simulink model "testbench_stateflow_20b"  (R2020b)
settings: Solver=VariableStepAuto  StartTime=0.0  StopTime=10  FixedStep=0.01  RelTol=1e-3  EnableMultiTasking=on
libraries: simulink x5
settings Model: Creator=Schneider  LastModifiedBy=60251
settings DataIOCC: LimitDataPoints=on  ReturnWorkspaceOutputs=off
settings OptimizationCC: LifeSpan=inf
settings DebuggingCC: AllowSymbolicDim=off  SFUnexpectedBacktrackingDiag=warning  SFNoUnconditionalDefaultTransitionDiag=warning  SFExecutionAtInitializationDiag=none  ArithmeticOperatorsInVariantConditions=warning
settings ModelReferenceCC: PropagateSignalLabelsOutOfModel=off
settings SFSimCC: SimUseLocalCustomCode=off  CustomCodeUndefinedFunction=UseInterfaceOnly
settings RTWCC: RTWUseLocalCustomCode=off
settings CodeAppCC: StateflowObjectComments=on
settings GRTTargetCC: TargetLangStandard=C89/C90 (ANSI)
settings ConfigComp: CovMetricSettings=dw  CovSaveCumulativeToWorkspaceVar=on  CovSaveSingleToWorkspaceVar=on  CovExternalEMLEnable=off

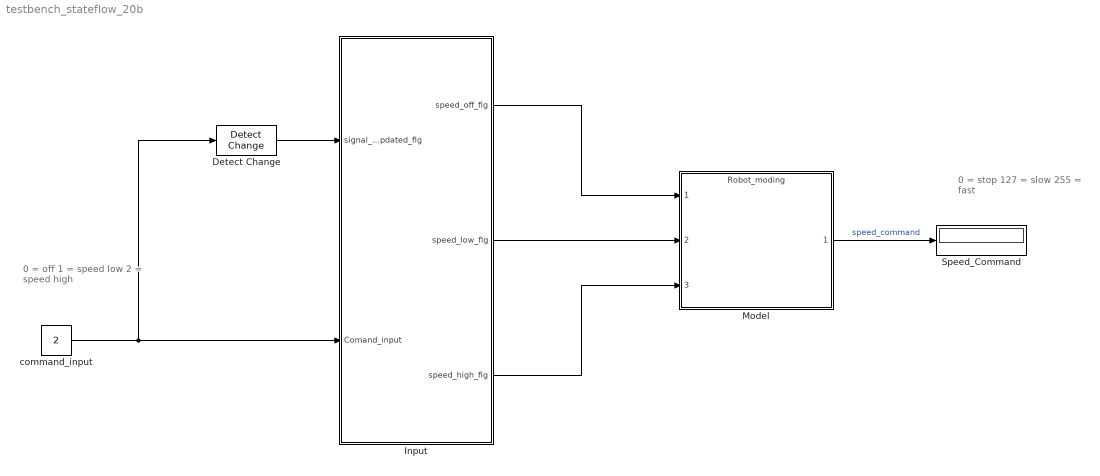
== system testbench_stateflow_20b ==
  note: 0     = stop
      | 127 = slow
      | 255 = fast
  note: 0 = off
      | 1 = speed low
      | 2 = speed high
  Detect Change : simulink/Logic and Bit Operations/Detect Change  vinit=0  OutDataTypeStr=boolean
  Input : Subsystem
  Model : ModelReference  ModelNameDialog=Robot_moding.slx  SimulationMode=Normal  ModelReferenceVersion=1.18
  Speed_Command : Display
  command_input : Constant  Value=2
  wires:
  Input/3(speed_high_flg) -> Model/3
  Input/2(speed_low_flg) -> Model/2
  Input/1(speed_off_flg) -> Model/1
  Detect Change/1 -> Input/1(" signal_updated_flg")
  command_input/1 -> Detect Change/1, Input/2(" Comand_input")
  Model/1 -> Speed_Command/1  "speed_command"

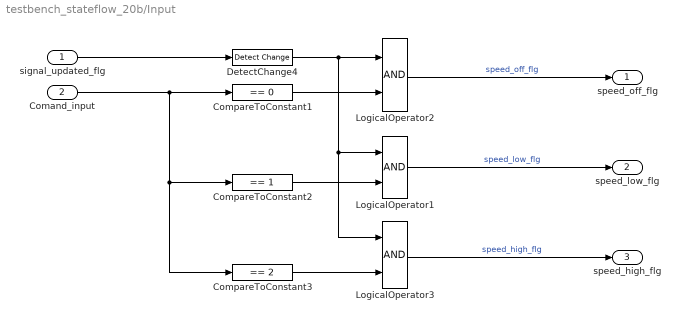
== system testbench_stateflow_20b/Input ==
  " signal_updated_flg" : Inport
  " Comand_input" : Inport  Port=2
  CompareToConstant1 : simulink/Logic and Bit Operations/Compare To Constant  relop===  const=0  OutDataTypeStr=boolean
  CompareToConstant2 : simulink/Logic and Bit Operations/Compare To Constant  relop===  const=1  OutDataTypeStr=boolean
  CompareToConstant3 : simulink/Logic and Bit Operations/Compare To Constant  relop===  const=2  OutDataTypeStr=boolean
  DetectChange4 : simulink/Logic and Bit Operations/Detect Change  vinit=0  OutDataTypeStr=boolean
  LogicalOperator1 : Logic  AllPortsSameDT=off  OutDataTypeStr=boolean
  LogicalOperator2 : Logic  AllPortsSameDT=off  OutDataTypeStr=boolean
  LogicalOperator3 : Logic  AllPortsSameDT=off  OutDataTypeStr=boolean
  speed_off_flg : Outport  OutDataTypeStr=boolean  VectorParamsAs1DForOutWhenUnconnected=off
  speed_low_flg : Outport  Port=2  OutDataTypeStr=boolean  VectorParamsAs1DForOutWhenUnconnected=off
  speed_high_flg : Outport  Port=3  OutDataTypeStr=boolean  VectorParamsAs1DForOutWhenUnconnected=off
  wires:
  LogicalOperator3/1 -> speed_high_flg/1  "speed_high_flg"
  LogicalOperator1/1 -> speed_low_flg/1  "speed_low_flg"
  LogicalOperator2/1 -> speed_off_flg/1  "speed_off_flg"
  " Comand_input"/1 -> CompareToConstant3/1, CompareToConstant2/1, CompareToConstant1/1
  CompareToConstant1/1 -> LogicalOperator2/2
  CompareToConstant3/1 -> LogicalOperator3/2
  CompareToConstant2/1 -> LogicalOperator1/2
  " signal_updated_flg"/1 -> DetectChange4/1
  DetectChange4/1 -> LogicalOperator3/1, LogicalOperator1/1, LogicalOperator2/1
